simulink model "Nav_inst1"  (R2021a)
settings: Solver=FixedStepAuto  StartTime=0.0  StopTime=timeFinal  FixedStep=timeStepMax  MaxStep=timeStepMax  RelTol=1e-3
model workspace (MAT data in the model file):
  x0 = 5
  y0 = 5
values from neighbouring files (symbols this model uses):
  a0 = x1_0    [run_Nav_inst1.m]
  a1 = x2_0    [run_Nav_inst1.m]
  b0 = v1_0    [run_Nav_inst1.m]
  b1 = v2_0    [run_Nav_inst1.m]
settings Model: SimulationMode=accelerator  Creator=amit  LastModifiedBy=amit
settings DataIOCC: ExternalInput=[x0, y0]

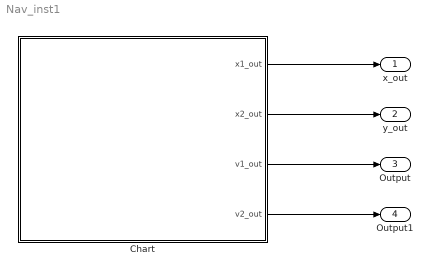
== system Nav_inst1 ==
  Chart : Stateflow chart  TreatAsAtomicUnit=on
  x_out : Outport  SignalName=x1Out
  y_out : Outport  Port=2  SignalName=x2Out
  Output : Outport  Port=3  SignalName=v1Out
  Output1 : Outport  Port=4  SignalName=v2Out
  wires:
  Chart/1(x1_out) -> x_out/1
  Chart/2(x2_out) -> y_out/1
  Chart/3(v1_out) -> Output/1
  Chart/4(v2_out) -> Output1/1

== stateflow chart Nav_inst1/Chart ==
  settings: updateMethod=CONTINUOUS  executeAtInitialization=1
  state loc9
    du:  % derivatives
    x1_dot = 1.0 * v1;
    x2_dot = 1.0 * v2;
    v1_dot = -1.2 * v1 + 0.1 * v2 + 0.1;
    v2_dot = 0.1 * v1 - 1.2 * v2 - 1.2;
    exit:
    x1_out=x1;
    x2_out=x2;
    v1_out=v1;
    v2_out=v2;
  state loc7
    du:
    x1_dot = 0;
    x2_dot = 0;
    v1_dot = 0;
    v2_dot = 0;
    exit:
    x1_out=x1;
    x2_out=x2;
    v1_out=v1;
    v2_out=v2;
  state loc8
    du:  % derivatives
    x1_dot = 1.0 * v1;
    x2_dot = 1.0 * v2;
    v1_dot = -1.2 * v1 + 0.1 * v2 + 1.2;
    v2_dot = 0.1 * v1 - 1.2 * v2 - 0.1;
    exit:
    x1_out=x1;
    x2_out=x2;
    v1_out=v1;
    v2_out=v2;
  state loc4
    du:  % derivatives
    x1_dot = 1.0 * v1;
    x2_dot = 1.0 * v2;
    v1_dot = -1.2 * v1 + 0.1 * v2 + 1.2;
    v2_dot = 0.1 * v1 - 1.2 * v2 - 0.1;
    exit:
    x1_out=x1;
    x2_out=x2;
    v1_out=v1;
    v2_out=v2;
  state loc5
    du:  % derivatives
    x1_dot = 1.0 * v1;
    x2_dot = 1.0 * v2;
    v1_dot = -1.2 * v1 + 0.1 * v2 + 1.2;
    v2_dot = 0.1 * v1 - 1.2 * v2 - 0.1;
    exit:
    x1_out=x1;
    x2_out=x2;
    v1_out=v1;
    v2_out=v2;
  state loc6
    du:  % derivatives
    x1_dot = 1.0 * v1;
    x2_dot = 1.0 * v2;
    v1_dot = -1.2 * v1 + 0.1 * v2 + 0.1;
    v2_dot = 0.1 * v1 - 1.2 * v2 - 1.2;
    exit:
    x1_out=x1;
    x2_out=x2;
    v1_out=v1;
    v2_out=v2;
  state loc3
    du:
    x1_dot = 0;
    x2_dot = 0;
    v1_dot = 0;
    v2_dot = 0;
    exit:
    x1_out=x1;
    x2_out=x2;
    v1_out=v1;
    v2_out=v2;
  state loc1
    du:  % derivatives
    x1_dot = 1.0 * v1;
    x2_dot = 1.0 * v2;
    v1_dot = -1.2 * v1 + 0.1 * v2 + 0.777821;
    v2_dot = 0.1 * v1 - 1.2 * v2 + 0.777821;
    exit:
    x1_out=x1;
    x2_out=x2;
    v1_out=v1;
    v2_out=v2;
  state loc2
    du:
    x1_dot = 1.0 * v1;
    x2_dot = 1.0 * v2;
    v1_dot = -1.2 * v1 + 0.1 * v2 + 0.777821;
    v2_dot = 0.1 * v1 - 1.2 * v2 + 0.777821;
    exit:
    x1_out=x1;
    x2_out=x2;
    v1_out=v1;
    v2_out=v2;
  loc8 -> loc8 [order 3] : [x1>=1 & x1<=2 & x2>=2 & x2<=3]{x1=x1; x2=x2; v1=v1; v2=v2;}
  loc7 -> loc7 : [x1>=0 & x1<=1 & x2>=2 & x2<=3]{x1=x1; x2=x2; v1=v1; v2=v2;}
  loc9 -> loc9 [order 3] : [x1>=2 & x1<=3 & x2>=2 & x2<=3]{x1=x1; x2=x2; v1=v1; v2=v2;}
  loc8 -> loc9 [order 2] : [x1>=2 & x2>=2 & x2<=3]{x1=x1; x2=x2; v1=v1; v2=v2;}
  loc8 -> loc7 [order 4] : [x1<1 & x2>=2 & x2<=3]{x1=x1; x2=x2; v1=v1; v2=v2;}
  loc9 -> loc8 [order 1] : [x1<2 & x2>=2 & x2<=3]{x1=x1; x2=x2; v1=v1; v2=v2;}
  loc9 -> loc6 [order 2] : [x1>=2 & x1<=3 & x2<2]{x1=x1; x2=x2; v1=v1; v2=v2;}
  loc6 -> loc9 [order 2] : [x1>=2 & x1<=3 & x2>=2]{x1=x1; x2=x2; v1=v1; v2=v2;}
  loc4 -> loc7 [order 1] : [x1>=0 & x1<=1 & x2>=2]{x1=x1; x2=x2; v1=v1; v2=v2;}
  loc5 -> loc8 [order 4] : [x1>=1 & x1<=2 & x2>=2]{x1=x1; x2=x2; v1=v1; v2=v2;}
  loc8 -> loc5 [order 1] : [x1>=1 & x1<=2 & x2<2]{x1=x1; x2=x2; v1=v1; v2=v2;}
  loc5 -> loc5 [order 5] : [x1>=1 & x1<=2 & x2>=1 & x2<=2]{x1=x1; x2=x2; v1=v1; v2=v2;}
  loc5 -> loc4 [order 1] : [x1<1 & x2>=1 & x2<=2]{x1=x1; x2=x2; v1=v1; v2=v2;}
  loc6 -> loc5 [order 3] : [x1<2 & x2>=1 & x2<=2]{x1=x1; x2=x2; v1=v1; v2=v2;}
  loc4 -> loc5 [order 2] : [x1>=1 & x2>=1 & x2<=2]{x1=x1; x2=x2; v1=v1; v2=v2;}
  loc4 -> loc4 [order 4] : [x1>=0 & x1<=1 & x2>=1 & x2<=2]{x1=x1; x2=x2; v1=v1; v2=v2;}
  loc5 -> loc6 [order 3] : [x1>=2 & x2>=1 & x2<=2]{x1=x1; x2=x2; v1=v1; v2=v2;}
  loc6 -> loc6 [order 4] : [x1>=2 & x1<=3 & x2>=1 & x2<=2]{x1=x1; x2=x2; v1=v1; v2=v2;}
  loc4 -> loc1 [order 3] : [x1>=0 & x1<=1 & x2<1]{x1=x1; x2=x2; v1=v1; v2=v2;}
  loc1 -> loc4 [order 2] : [x1>=0 & x1<=1 & x2>=1]{x1=x1; x2=x2; v1=v1; v2=v2;}
  loc6 -> loc3 [order 1] : [x1>=2 & x1<=3 & x2<=1]{x1=x1; x2=x2; v1=v1; v2=v2;}
  loc2 -> loc5 [order 2] : [x1>=1 & x1<=2 & x2>=1]{x1=x1; x2=x2; v1=v1; v2=v2;}
  loc5 -> loc2 [order 2] : [x1>=1 & x1<=2 & x2<1]{x1=x1; x2=x2; v1=v1; v2=v2;}
  loc2 -> loc1 [order 3] : [x1<1 & x2>=0 & x2<=1]{x1=x1; x2=x2; v1=v1; v2=v2;}
  loc1 -> loc1 [order 3] : [x1>=0 & x1<=1 & x2>=0 & x2<=1]{x1=x1; x2=x2; v1=v1; v2=v2;}
  loc2 -> loc3 [order 1] : [x1>=2 & x2>=0 & x2<=1]{x1=x1; x2=x2; v1=v1; v2=v2;}
  loc1 -> loc2 [order 1] : [x1>=1 & x2>=0 & x2<=1]{x1=x1; x2=x2; v1=v1; v2=v2;}
  loc3 -> loc3 : [x1>=2 & x1<=3 & x2>=0 & x2<=1]{x1=x1; x2=x2; v1=v1; v2=v2;}
  (default) -> loc1 : {x1=a0; x2=a1; v1=b0; v2=b1;}
  loc2 -> loc2 [order 4] : [x1>=1 & x1<=2 & x2>=0 & x2<=1]{x1=x1; x2=x2; v1=v1; v2=v2;}
  data: a0 parameter; a1 parameter; b0 parameter; b1 parameter; x1_out output; x2_out output; v1_out output; v2_out output; x1 local; x2 local; v1 local; v2 local
  data x1 settings: updateMethod=SF_CONTINUOUS_TIME_DATA
  data x2 settings: updateMethod=SF_CONTINUOUS_TIME_DATA
  data v1 settings: updateMethod=SF_CONTINUOUS_TIME_DATA
  data v2 settings: updateMethod=SF_CONTINUOUS_TIME_DATA
